simulink model "one_actuator"  (Simulink 10.0)
settings: Solver=FixedStepAuto  StartTime=0.0  StopTime=60  FixedStep=fixedStep  MaxStep=0.2  RelTol=1e-3
values from neighbouring files (symbols this model uses):
  dc = (l+r)/2    (= 5)    [tempModel.m]
  dx = (xmax-xmin)/(N-1)    (= 0.05)    [temperatureParametersInitWindow.m]
  xx = xmin:dx:xmax    [temperatureParametersInitWindow.m]
undefined symbols (not defined in the file or in its folder): parameters1, x01
settings Model: Creator=lixuansong  LastModifiedBy=Ozgur Ozmen
settings DataIOCC: SaveOutput=off  SignalLogging=off  DSMLogging=off
settings OptimizationCC: LifeSpan=auto
settings DebuggingCC: UnderspecifiedInitializationDetection=Simplified  MergeDetectMultiDrivingBlocksExec=error  SFUnexpectedBacktrackingDiag=error  SFNoUnconditionalDefaultTransitionDiag=error  SFExecutionAtInitializationDiag=warning  ArithmeticOperatorsInVariantConditions=error
settings HardwareCC: ProdBitPerPointer=64  ProdBitPerSizeT=64  ProdBitPerPtrDiffT=64  ProdLargestAtomicFloat=Float  ProdIntDivRoundTo=Zero  ProdEndianess=LittleEndian  ProdWordSize=64  ProdHWDeviceType=Intel->x86-64 (Windows64)
settings ModelReferenceCC: PropagateSignalLabelsOutOfModel=on
settings SFSimCC: SimUseLocalCustomCode=on  CustomCodeUndefinedFunction=FilterOut
settings RTWCC: RTWUseLocalCustomCode=on
settings CodeAppCC: StateflowObjectComments=off
settings GRTTargetCC: TargetLangStandard=C99 (ISO)  CombineOutputUpdateFcns=on  GRTInterface=off
settings ConfigComp: CovMetricSettings=dwe  CovHtmlReporting=off  CovSaveCumulativeToWorkspaceVar=off  CovSaveSingleToWorkspaceVar=off

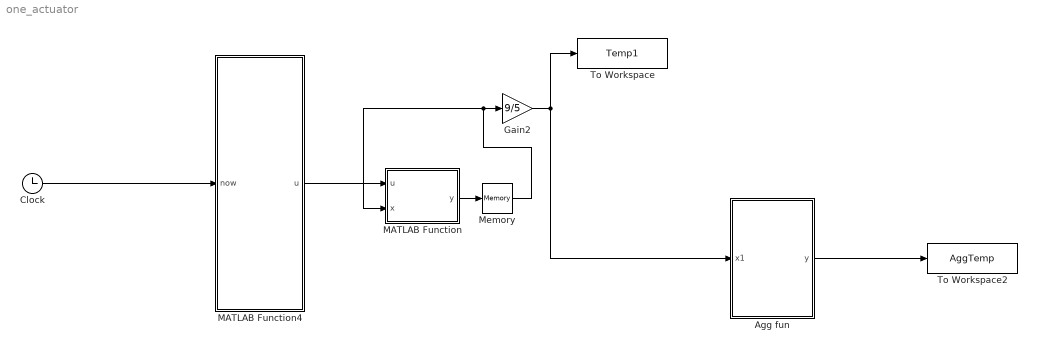
== system one_actuator ==
  Agg fun : MATLAB Function  TreatAsAtomicUnit=on
  Clock : Clock
  Gain2 : Gain  Gain=9/5
  MATLAB Function : MATLAB Function  TreatAsAtomicUnit=on
  MATLAB Function4 : MATLAB Function  TreatAsAtomicUnit=on
  Memory : Memory  InitialCondition=x01
  To Workspace : ToWorkspace  VariableName=Temp1  SampleTime=-1
  To Workspace2 : ToWorkspace  VariableName=AggTemp  SampleTime=-1
  wires:
  MATLAB Function/1(y) -> Memory/1
  Memory/1 -> MATLAB Function/2(x), Gain2/1
  MATLAB Function4/1(u) -> MATLAB Function/1(u)
  Clock/1 -> MATLAB Function4/1(now)
  Agg fun/1(y) -> To Workspace2/1
  Gain2/1 -> To Workspace/1, Agg fun/1(x1)

== matlab function MATLAB Function ==
  data: u input double; y output double; x input double; parameters1 parameter double; xx parameter double
function y = coffeeMaker(u,x,parameters1, xx)




tL=parameters1(:,1);
tR=parameters1(:,2);
lambda=parameters1(:,3);


    temp1=x;
    
        
    
             for i = 1:length(xx) % for space steps
                if i == 1
                    temp1(i) = u*tL;
              %     temp1(i) = tL;
                elseif i == length(xx)
                    temp1(i) = tR;
                else 
                    temp1(i) = temp1(i)+lambda*(temp1(i+1)-2*temp1(i)+temp1(i-1));
                end
            end
y = temp1;

== matlab function Agg fun ==
  data: x1 input double; y output double; dx parameter double; dc parameter double
function y = agg(x1,dx, dc)

disCoffee=getDisPos(dc,dx);

y = x1(disCoffee+1);

== matlab function MATLAB Function4 ==
  data: u output double; now input double; timeCoffee parameter double
function u = controlCoffee(now,timeCoffee)
if now>=0 && now<=timeCoffee
    u=1;
else
    u=0;
end
